simulink model "verify_Ventilation_mdl"  (R2018b)
settings: Solver=VariableStepDiscrete  StartTime=0  StopTime=100  MaxStep=5  RelTol=1e-3  EnableMultiTasking=on
libraries: carnot x2, simulink x1
settings Model: Creator=drhf  LastModifiedBy=drhf
settings DataIOCC: SaveFormat=Array  SignalLoggingSaveFormat=ModelDataLogs
settings OptimizationCC: ExpressionDepthLimit=2147483647  LifeSpan=inf
settings DebuggingCC: UnderspecifiedInitializationDetection=Classic  MergeDetectMultiDrivingBlocksExec=none  SolverPrmCheckMsg=warning  FcnCallInpInsideContextMsg=warning  StateNameClashWarn=warning  SFUnexpectedBacktrackingDiag=warning  SFNoUnconditionalDefaultTransitionDiag=warning  SFExecutionAtInitializationDiag=none
settings HardwareCC: ProdBitPerPointer=32  ProdBitPerSizeT=32  ProdBitPerPtrDiffT=32  ProdLargestAtomicFloat=None  ProdIntDivRoundTo=Undefined  ProdEndianess=Unspecified  ProdWordSize=32  ProdHWDeviceType=32-bit Generic
settings ModelReferenceCC: PropagateSignalLabelsOutOfModel=off
settings SFSimCC: SimUseLocalCustomCode=off
settings RTWCC: RTWUseLocalCustomCode=off
settings CodeAppCC: StateflowObjectComments=on
settings GRTTargetCC: TargetLangStandard=C89/C90 (ANSI)  GeneratePreprocessorConditionals=Disable all  CombineOutputUpdateFcns=off  GRTInterface=on
settings ConfigComp: CovMetricSettings=dw  CovHtmlReporting=on  CovSaveCumulativeToWorkspaceVar=on  CovSaveSingleToWorkspaceVar=on  CovExternalEMLEnable=off

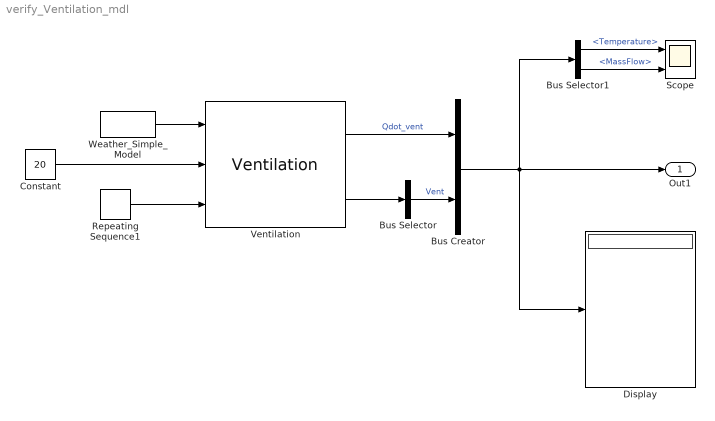
== system verify_Ventilation_mdl ==
  Bus Creator : BusCreator  Inputs=2
  Bus Selector : BusSelector  OutputSignals=Temperature,MassFlow,Pressure,FluidMix  OutputAsBus=on
  Bus Selector1 : BusSelector  OutputSignals=Vent.Temperature,Vent.MassFlow
  Constant : Constant  Value=20
  Display : Display
  Repeating Sequence1 : simulink/Sources/Repeating Sequence  rep_seq_t=[0 20 30 60 70 100]  rep_seq_y="[0  0  1   1   0   0]"
  Scope : Scope  NumInputPorts=2
  Ventilation : carnot/Source/Ventilation/Ventilation  Ahabit=50  Hroom=2  vent=0.6  rec=0.6  ppmCO2=400  ppmVOC=0  alpha=10  H=1  W=1  Nwin=1
      settings: SourceProductName=Carnot
  Weather_Simple_Model : carnot/Weather/Weather_Simple_Model  Ibn=900  Idg=100  tamb=0  deltaTsky=-6  rh=50  precip="10e-3/24/3600           % 10 mm in 24 h"  cloud=0.125  p=1013e2  vw=1  wdir=270  lat=60  colangle=0  colazi=0  colrot=0
      settings: SourceProductName=Carnot
  Out1 : Outport
  wires:
  Ventilation/1 -> Bus Creator/1  "Qdot_vent"
  Constant/1 -> Ventilation/2
  Repeating Sequence1/1 -> Ventilation/3
  Bus Creator/1 -> Display/1, Bus Selector1/1, Out1/1
  Ventilation/2 -> Bus Selector/1
  Bus Selector/1 -> Bus Creator/2  "Vent"
  Weather_Simple_Model/1 -> Ventilation/1
  Bus Selector1/1 -> Scope/1  "<Temperature>"
  Bus Selector1/2 -> Scope/2  "<MassFlow>"
